simulink model "n98tot98reg57neu"  (R2023b)
settings: Solver=VariableStepAuto  StartTime=0.0  StopTime=10.0  RelTol=1e-3
libraries: neural x63
(part 2 of 3)

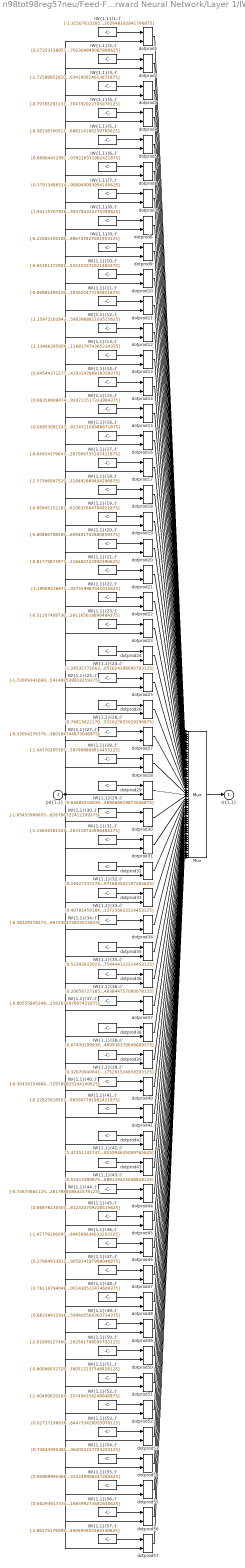
== system n98tot98reg57neu/Feed-Forward Neural Network/Layer 1/IW{1,1} ==
  "pd{1,1}" : Inport  PortDimensions=7
      mask Display: e = 0.06;c1 = [120 230 180]/255;c2 = ([120 230 180]+0)/(256+128);c3 = ([120 230 180]+128)/(256+128);patch([0 1 1 0],[0 0 1 1],c1);patch([0 1 1 1-e 1-e 0+e],[0 0 1 1-e 0+e 0+e],c2);patch([0 0 1 1-e 0+e 0+e],[0 1 1 1-e 1-e 0+e],c3);plot([0 1 1 0 0],[0 0 1 1 0]);
  "IW{1,1}(1,:)'" : Constant  Value=[-1.31507613281385449255367348087020218372344970703125;-0.3434268124643267139362023954163305461406707763671875;-0.4055668892280188675414365206961520016193389892578125;-0.58108307602678055392431133441277779638767242431640625;-1.2280217354284930220131855094223283231258392333984375;1.168197906116284823241358026280067861080169677734375;-0.55694114732430921588246519604581408202648162841796875]
      mask Display: e = 0.06;c1 = [120 150 230]/255;c2 = ([120 150 230]+0)/383;c3 = ([120 150 230]+128)/383;patch([0 1 1 0],[0 0 1 1],c1);patch([0 1 1 1-e 1-e 0+e],[0 0 1 1-e 0+e 0+e],c2);patch([0 0 1 1-e 0+e 0+e],[0 1 1 1-e 1-e 0+e],c3);plot([0 1 1 0 0],[0 0 1 1 0]);disp('Weights');
  "IW{1,1}(10,:)'" : Constant  Value=[-0.65301172901308179863377745277830399572849273681640625;0.557094329633779583588193418108858168125152587890625;-0.84973696392753306216860664790146984159946441650390625;-0.632442901627863651725647287094034254550933837890625;0.99820207808413707883943288834416307508945465087890625;-0.8724231506525537138685422178241424262523651123046875;0.76560493245783245441771214245818555355072021484375]
      mask Display: e = 0.06;c1 = [120 150 230]/255;c2 = ([120 150 230]+0)/383;c3 = ([120 150 230]+128)/383;patch([0 1 1 0],[0 0 1 1],c1);patch([0 1 1 1-e 1-e 0+e],[0 0 1 1-e 0+e 0+e],c2);patch([0 0 1 1-e 0+e 0+e],[0 1 1 1-e 1-e 0+e],c3);plot([0 1 1 0 0],[0 0 1 1 0]);disp('Weights');
  "IW{1,1}(11,:)'" : Constant  Value=[-0.06985499326512305262593116594871389679610729217529296875;-1.55742226767316171986976769403554499149322509765625;0.61111449383935878554297005393891595304012298583984375;-0.0637891933373135600060521710474858991801738739013671875;1.12246939262949130267088548862375319004058837890625;-1.345762851134290283283689859672449529170989990234375;0.95876871436280175498012567913974635303020477294921875]
      mask Display: e = 0.06;c1 = [120 150 230]/255;c2 = ([120 150 230]+0)/383;c3 = ([120 150 230]+128)/383;patch([0 1 1 0],[0 0 1 1],c1);patch([0 1 1 1-e 1-e 0+e],[0 0 1 1-e 0+e 0+e],c2);patch([0 0 1 1-e 0+e 0+e],[0 1 1 1-e 1-e 0+e],c3);plot([0 1 1 0 0],[0 0 1 1 0]);disp('Weights');
  "IW{1,1}(12,:)'" : Constant  Value=[2.159721626433666497035801512538455426692962646484375;-1.1313148038546676499294107998139224946498870849609375;-0.66185085994261905195656936484738253057003021240234375;1.6817370764954191475482048190315254032611846923828125;-0.93077989098894853281507266729022376239299774169921875;-1.173094338058920715894828390446491539478302001953125;1.2382244436054552494397285045124590396881103515625]
      mask Display: e = 0.06;c1 = [120 150 230]/255;c2 = ([120 150 230]+0)/383;c3 = ([120 150 230]+128)/383;patch([0 1 1 0],[0 0 1 1],c1);patch([0 1 1 1-e 1-e 0+e],[0 0 1 1-e 0+e 0+e],c2);patch([0 0 1 1-e 0+e 0+e],[0 1 1 1-e 1-e 0+e],c3);plot([0 1 1 0 0],[0 0 1 1 0]);disp('Weights');
  "IW{1,1}(13,:)'" : Constant  Value=[2.134962850094378250531690355273894965648651123046875;0.1810173913040981352740033116788254119455814361572265625;0.1268442563962487723561167740626842714846134185791015625;2.077238884587504497147847359883598983287811279296875;-0.03626682177452443534004800085313036106526851654052734375;-1.7725082910032003979949877248145639896392822265625;0.597079894289870960477628614171408116817474365234375]
      mask Display: e = 0.06;c1 = [120 150 230]/255;c2 = ([120 150 230]+0)/383;c3 = ([120 150 230]+128)/383;patch([0 1 1 0],[0 0 1 1],c1);patch([0 1 1 1-e 1-e 0+e],[0 0 1 1-e 0+e 0+e],c2);patch([0 0 1 1-e 0+e 0+e],[0 1 1 1-e 1-e 0+e],c3);plot([0 1 1 0 0],[0 0 1 1 0]);disp('Weights');
  "IW{1,1}(14,:)'" : Constant  Value=[0.945442711778084809992606096784584224224090576171875;-0.0565352619944564926957042416688636876642704010009765625;0.91502969793743405002572899320512078702449798583984375;-1.3291403247332258530377657734788954257965087890625;-0.71424304769140800619453557374072261154651641845703125;1.440252227385283134708515717647969722747802734375;-0.31626437150536046427617975496104918420314788818359375]
      mask Display: e = 0.06;c1 = [120 150 230]/255;c2 = ([120 150 230]+0)/383;c3 = ([120 150 230]+128)/383;patch([0 1 1 0],[0 0 1 1],c1);patch([0 1 1 1-e 1-e 0+e],[0 0 1 1-e 0+e 0+e],c2);patch([0 0 1 1-e 0+e 0+e],[0 1 1 1-e 1-e 0+e],c3);plot([0 1 1 0 0],[0 0 1 1 0]);disp('Weights');
  "IW{1,1}(15,:)'" : Constant  Value=[0.9635960847448152843952584589715115725994110107421875;0.09980816968357765495145628165118978358805179595947265625;-0.50121653240937102946617187626543454825878143310546875;-1.919415213736128666965896627516485750675201416015625;0.47845586929562278211136572281247936189174652099609375;0.941812528879230281830814419663511216640472412109375;-0.86980200940910579188170004272251389920711517333984375]
      mask Display: e = 0.06;c1 = [120 150 230]/255;c2 = ([120 150 230]+0)/383;c3 = ([120 150 230]+128)/383;patch([0 1 1 0],[0 0 1 1],c1);patch([0 1 1 1-e 1-e 0+e],[0 0 1 1-e 0+e 0+e],c2);patch([0 0 1 1-e 0+e 0+e],[0 1 1 1-e 1-e 0+e],c3);plot([0 1 1 0 0],[0 0 1 1 0]);disp('Weights');
  "IW{1,1}(16,:)'" : Constant  Value=[0.0085309114777282722685836091613964526914060115814208984375;0.76963678008214742032322419618139974772930145263671875;0.633935904479372869246844857116229832172393798828125;-0.459413204321313883848887371641467325389385223388671875;-2.435905516746778243231119631673209369182586669921875;0.77012835966411830046496334034600295126438140869140625;-0.484808047650836015929343147945473901927471160888671875]
      mask Display: e = 0.06;c1 = [120 150 230]/255;c2 = ([120 150 230]+0)/383;c3 = ([120 150 230]+128)/383;patch([0 1 1 0],[0 0 1 1],c1);patch([0 1 1 1-e 1-e 0+e],[0 0 1 1-e 0+e 0+e],c2);patch([0 0 1 1-e 0+e 0+e],[0 1 1 1-e 1-e 0+e],c3);plot([0 1 1 0 0],[0 0 1 1 0]);disp('Weights');
  "IW{1,1}(17,:)'" : Constant  Value=[-0.64954379643572435210074900169274769723415374755859375;0.5455804121247702642705235120956785976886749267578125;-1.5634615988825759647085078540840186178684234619140625;-0.84212075753120385623873289659968577325344085693359375;0.5360456525378729519815124149317853152751922607421875;-1.4042701008338334123237700623576529324054718017578125;0.21773378780089636119754459286923520267009735107421875]
      mask Display: e = 0.06;c1 = [120 150 230]/255;c2 = ([120 150 230]+0)/383;c3 = ([120 150 230]+128)/383;patch([0 1 1 0],[0 0 1 1],c1);patch([0 1 1 1-e 1-e 0+e],[0 0 1 1-e 0+e 0+e],c2);patch([0 0 1 1-e 0+e 0+e],[0 1 1 1-e 1-e 0+e],c3);plot([0 1 1 0 0],[0 0 1 1 0]);disp('Weights');
  "IW{1,1}(18,:)'" : Constant  Value=[-1.575660475296334350758797882008366286754608154296875;1.8425130461237986256861631773062981665134429931640625;0.781192060847692548719578553573228418827056884765625;1.09892397924112827922726864926517009735107421875;-0.976082267335859565804412341094575822353363037109375;-0.6852967127598470487015447361045517027378082275390625;-0.71498884111504767968625628782319836318492889404296875]
      mask Display: e = 0.06;c1 = [120 150 230]/255;c2 = ([120 150 230]+0)/383;c3 = ([120 150 230]+128)/383;patch([0 1 1 0],[0 0 1 1],c1);patch([0 1 1 1-e 1-e 0+e],[0 0 1 1-e 0+e 0+e],c2);patch([0 0 1 1-e 0+e 0+e],[0 1 1 1-e 1-e 0+e],c3);plot([0 1 1 0 0],[0 0 1 1 0]);disp('Weights');
  "IW{1,1}(19,:)'" : Constant  Value=[-0.9594515218334020989487953556817956268787384033203125;-0.48829379470511657945763772659120149910449981689453125;0.4757457278855803384232103780959732830524444580078125;0.9005439753059005791868685264489613473415374755859375;-1.0185701269266511648226014585816301405429840087890625;-1.4773529160647649316473462022258900105953216552734375;-0.726355990881138335879541045869700610637664794921875]
      mask Display: e = 0.06;c1 = [120 150 230]/255;c2 = ([120 150 230]+0)/383;c3 = ([120 150 230]+128)/383;patch([0 1 1 0],[0 0 1 1],c1);patch([0 1 1 1-e 1-e 0+e],[0 0 1 1-e 0+e 0+e],c2);patch([0 0 1 1-e 0+e 0+e],[0 1 1 1-e 1-e 0+e],c3);plot([0 1 1 0 0],[0 0 1 1 0]);disp('Weights');
  "IW{1,1}(2,:)'" : Constant  Value=[0.272531380514197840714274434503749944269657135009765625;1.0968943883890844848139067835290916264057159423828125;-0.34251944384713095548278261048835702240467071533203125;-0.874463157238554611438985375571064651012420654296875;0.9507141217692856027809966690256260335445404052734375;-0.24034301968930471549157346089486964046955108642578125;1.6368628806959615307192734690033830702304840087890625]
      mask Display: e = 0.06;c1 = [120 150 230]/255;c2 = ([120 150 230]+0)/383;c3 = ([120 150 230]+128)/383;patch([0 1 1 0],[0 0 1 1],c1);patch([0 1 1 1-e 1-e 0+e],[0 0 1 1-e 0+e 0+e],c2);patch([0 0 1 1-e 0+e 0+e],[0 1 1 1-e 1-e 0+e],c3);plot([0 1 1 0 0],[0 0 1 1 0]);disp('Weights');
  "IW{1,1}(20,:)'" : Constant  Value=[-0.8088679858537386468952945506316609680652618408203125;0.11185596548077370027129973095725290477275848388671875;1.026306998840350814816702040843665599822998046875;-0.2193307597737976510909874150456744246184825897216796875;0.96539895136091613547790757365874014794826507568359375;-1.611240681871787483459002032759599387645721435546875;0.1380372426352799164472884285714826546609401702880859375]
      mask Display: e = 0.06;c1 = [120 150 230]/255;c2 = ([120 150 230]+0)/383;c3 = ([120 150 230]+128)/383;patch([0 1 1 0],[0 0 1 1],c1);patch([0 1 1 1-e 1-e 0+e],[0 0 1 1-e 0+e 0+e],c2);patch([0 0 1 1-e 0+e 0+e],[0 1 1 1-e 1-e 0+e],c3);plot([0 1 1 0 0],[0 0 1 1 0]);disp('Weights');
  "IW{1,1}(21,:)'" : Constant  Value=[-0.8177987397310102490877170566818676888942718505859375;-0.3905060399106281554537645206437446177005767822265625;0.11055547284934041929460590836242772638797760009765625;0.1052993247470589144310082474476075731217861175537109375;-1.2126110654717712211692060009227134287357330322265625;0.607129439275836180200940361828543245792388916015625;-2.50415210712362412692755242460407316684722900390625]
      mask Display: e = 0.06;c1 = [120 150 230]/255;c2 = ([120 150 230]+0)/383;c3 = ([120 150 230]+128)/383;patch([0 1 1 0],[0 0 1 1],c1);patch([0 1 1 1-e 1-e 0+e],[0 0 1 1-e 0+e 0+e],c2);patch([0 0 1 1-e 0+e 0+e],[0 1 1 1-e 1-e 0+e],c3);plot([0 1 1 0 0],[0 0 1 1 0]);disp('Weights');
  "IW{1,1}(22,:)'" : Constant  Value=[1.19089226971850781211514913593418896198272705078125;1.45385364381177151216206766548566520214080810546875;-0.601277074598317806675140673178248107433319091796875;-0.475071026226747961107577111761202104389667510986328125;1.1590060828883947952050448293448425829410552978515625;-0.223577539094418853427015392298926599323749542236328125;0.52854958185949441062945197700173594057559967041015625]
      mask Display: e = 0.06;c1 = [120 150 230]/255;c2 = ([120 150 230]+0)/383;c3 = ([120 150 230]+128)/383;patch([0 1 1 0],[0 0 1 1],c1);patch([0 1 1 1-e 1-e 0+e],[0 0 1 1-e 0+e 0+e],c2);patch([0 0 1 1-e 0+e 0+e],[0 1 1 1-e 1-e 0+e],c3);plot([0 1 1 0 0],[0 0 1 1 0]);disp('Weights');
  "IW{1,1}(23,:)'" : Constant  Value=[-0.51107408730064118884683921351097524166107177734375;-0.69542516098775897237516119275824166834354400634765625;-1.4905003550878583862271398174925707280635833740234375;1.0412183770694818374380474779172800481319427490234375;-0.858888834537086420795048979925923049449920654296875;0.126966453545523716428533589350990951061248779296875;-0.879111162983166050111094591557048261165618896484375]
      mask Display: e = 0.06;c1 = [120 150 230]/255;c2 = ([120 150 230]+0)/383;c3 = ([120 150 230]+128)/383;patch([0 1 1 0],[0 0 1 1],c1);patch([0 1 1 1-e 1-e 0+e],[0 0 1 1-e 0+e 0+e],c2);patch([0 0 1 1-e 0+e 0+e],[0 1 1 1-e 1-e 0+e],c3);plot([0 1 1 0 0],[0 0 1 1 0]);disp('Weights');
  "IW{1,1}(24,:)'" : Constant  Value=[1.2453577166389904196108773248852230608463287353515625;-0.242279955231003818472146349449758417904376983642578125;-0.6152732028289682464361476377234794199466705322265625;-0.52848261741762225796037455438636243343353271484375;-1.3356713480763762191827481728978455066680908203125;-0.7798150291085292895587599559803493320941925048828125;1.316557903300858090034353153896518051624298095703125]
      mask Display: e = 0.06;c1 = [120 150 230]/255;c2 = ([120 150 230]+0)/383;c3 = ([120 150 230]+128)/383;patch([0 1 1 0],[0 0 1 1],c1);patch([0 1 1 1-e 1-e 0+e],[0 0 1 1-e 0+e 0+e],c2);patch([0 0 1 1-e 0+e 0+e],[0 1 1 1-e 1-e 0+e],c3);plot([0 1 1 0 0],[0 0 1 1 0]);disp('Weights');
  "IW{1,1}(25,:)'" : Constant  Value=[-1.720093416906787187059535426669754087924957275390625;-1.1755779750190813448540438912459649145603179931640625;-0.273381324463259745005672129991580732166767120361328125;0.92851119014197058820769825615570880472660064697265625;0.78830859911427586528276378885493613779544830322265625;0.53710877686837321665080935417790897190570831298828125;-0.0931050198316623889294163518570712767541408538818359375]
      mask Display: e = 0.06;c1 = [120 150 230]/255;c2 = ([120 150 230]+0)/383;c3 = ([120 150 230]+128)/383;patch([0 1 1 0],[0 0 1 1],c1);patch([0 1 1 1-e 1-e 0+e],[0 0 1 1-e 0+e 0+e],c2);patch([0 0 1 1-e 0+e 0+e],[0 1 1 1-e 1-e 0+e],c3);plot([0 1 1 0 0],[0 0 1 1 0]);disp('Weights');
  "IW{1,1}(26,:)'" : Constant  Value=[0.7681562217053945484934729392989538609981536865234375;1.3209871255882330576270078381639905273914337158203125;-0.495847608712504717143332300111069343984127044677734375;-0.768492213819274905262091124313883483409881591796875;1.4607032300264208846130031815846450626850128173828125;1.4314160847875883053603729422320611774921417236328125;0.63011690839067202585255245139705948531627655029296875]
      mask Display: e = 0.06;c1 = [120 150 230]/255;c2 = ([120 150 230]+0)/383;c3 = ([120 150 230]+128)/383;patch([0 1 1 0],[0 0 1 1],c1);patch([0 1 1 1-e 1-e 0+e],[0 0 1 1-e 0+e 0+e],c2);patch([0 0 1 1-e 0+e 0+e],[0 1 1 1-e 1-e 0+e],c3);plot([0 1 1 0 0],[0 0 1 1 0]);disp('Weights');
  "IW{1,1}(27,:)'" : Constant  Value=[-0.330542763766594027696754665157641284167766571044921875;1.4209623056183582345823879222734831273555755615234375;-1.3540278759723431978301277922582812607288360595703125;1.239950698517690685918068993487395346164703369140625;0.244622420985858901598675174682284705340862274169921875;-0.69335046389705023983651699381880462169647216796875;0.04286899583435747895787670813660952262580394744873046875]
      mask Display: e = 0.06;c1 = [120 150 230]/255;c2 = ([120 150 230]+0)/383;c3 = ([120 150 230]+128)/383;patch([0 1 1 0],[0 0 1 1],c1);patch([0 1 1 1-e 1-e 0+e],[0 0 1 1-e 0+e 0+e],c2);patch([0 0 1 1-e 0+e 0+e],[0 1 1 1-e 1-e 0+e],c3);plot([0 1 1 0 0],[0 0 1 1 0]);disp('Weights');
  "IW{1,1}(28,:)'" : Constant  Value=[-1.44370205397184481199701622244901955127716064453125;0.483062098703527009746494513819925487041473388671875;0.325262798677855291540339521816349588334560394287109375;1.87353161972341819563325771014206111431121826171875;-0.469898365036419407569923123446642421185970306396484375;-0.52795627331928962622242806901340372860431671142578125;-0.6150982768929271760072197139379568397998809814453125]
      mask Display: e = 0.06;c1 = [120 150 230]/255;c2 = ([120 150 230]+0)/383;c3 = ([120 150 230]+128)/383;patch([0 1 1 0],[0 0 1 1],c1);patch([0 1 1 1-e 1-e 0+e],[0 0 1 1-e 0+e 0+e],c2);patch([0 0 1 1-e 0+e 0+e],[0 1 1 1-e 1-e 0+e],c3);plot([0 1 1 0 0],[0 0 1 1 0]);disp('Weights');
  "IW{1,1}(29,:)'" : Constant  Value=[0.64685516039214252526079462768393568694591522216796875;-0.7133517745537172327630059953662566840648651123046875;-1.1162505593597875641620476017124019563198089599609375;1.4296859613759911322716789072728715837001800537109375;-1.673504671100669582983755390159785747528076171875;-0.2356418802824417346730712097269133664667606353759765625;0.1731214195331098604224706605236860923469066619873046875]
      mask Display: e = 0.06;c1 = [120 150 230]/255;c2 = ([120 150 230]+0)/383;c3 = ([120 150 230]+128)/383;patch([0 1 1 0],[0 0 1 1],c1);patch([0 1 1 1-e 1-e 0+e],[0 0 1 1-e 0+e 0+e],c2);patch([0 0 1 1-e 0+e 0+e],[0 1 1 1-e 1-e 0+e],c3);plot([0 1 1 0 0],[0 0 1 1 0]);disp('Weights');
  "IW{1,1}(3,:)'" : Constant  Value=[-1.7258895161045704202962269846466369926929473876953125;-0.96905544802317578056971569822053425014019012451171875;-0.2467907702150093085524673597319633699953556060791015625;0.620713226509980398049037830787710845470428466796875;-0.58216038095865296764230834014597348868846893310546875;0.8234144012332003104148725469713099300861358642578125;0.69431564257952060881251554746995680034160614013671875]
      mask Display: e = 0.06;c1 = [120 150 230]/255;c2 = ([120 150 230]+0)/383;c3 = ([120 150 230]+128)/383;patch([0 1 1 0],[0 0 1 1],c1);patch([0 1 1 1-e 1-e 0+e],[0 0 1 1-e 0+e 0+e],c2);patch([0 0 1 1-e 0+e 0+e],[0 1 1 1-e 1-e 0+e],c3);plot([0 1 1 0 0],[0 0 1 1 0]);disp('Weights');
  "IW{1,1}(30,:)'" : Constant  Value=[-1.05455966655188593250613848795183002948760986328125;0.627223375235642865987983896047808229923248291015625;0.12537337491597810856802652779151685535907745361328125;0.2444653558883956023795036571755190379917621612548828125;-0.66100938577782974991947639864520169794559478759765625;-0.360249769337874337082894271588884294033050537109375;1.6012452229692220040391248403466306626796722412109375]
      mask Display: e = 0.06;c1 = [120 150 230]/255;c2 = ([120 150 230]+0)/383;c3 = ([120 150 230]+128)/383;patch([0 1 1 0],[0 0 1 1],c1);patch([0 1 1 1-e 1-e 0+e],[0 0 1 1-e 0+e 0+e],c2);patch([0 0 1 1-e 0+e 0+e],[0 1 1 1-e 1-e 0+e],c3);plot([0 1 1 0 0],[0 0 1 1 0]);disp('Weights');
  "IW{1,1}(31,:)'" : Constant  Value=[-1.1563458134754280859368691380950622260570526123046875;-0.93459383751556490693701562122441828250885009765625;-1.3360775871392422953221057468908838927745819091796875;0.0993024254056518451694302029864047653973102569580078125;0.00133754034631904106245059438151656650006771087646484375;-0.67390772930921460925901556038297712802886962890625;-1.3895944435588647447588073191582225263118743896484375]
      mask Display: e = 0.06;c1 = [120 150 230]/255;c2 = ([120 150 230]+0)/383;c3 = ([120 150 230]+128)/383;patch([0 1 1 0],[0 0 1 1],c1);patch([0 1 1 1-e 1-e 0+e],[0 0 1 1-e 0+e 0+e],c2);patch([0 0 1 1-e 0+e 0+e],[0 1 1 1-e 1-e 0+e],c3);plot([0 1 1 0 0],[0 0 1 1 0]);disp('Weights');
  "IW{1,1}(32,:)'" : Constant  Value=[0.164273372784759341680427269238862209022045135498046875;0.33065648688842308455804186451132409274578094482421875;-1.0794971677089122419346267633954994380474090576171875;-0.7715801043565042593996849973336793482303619384765625;2.13032359300715246064328312058933079242706298828125;-0.67381390592311607434794495929963886737823486328125;-0.416767412004134973901869898327277041971683502197265625]
      mask Display: e = 0.06;c1 = [120 150 230]/255;c2 = ([120 150 230]+0)/383;c3 = ([120 150 230]+128)/383;patch([0 1 1 0],[0 0 1 1],c1);patch([0 1 1 1-e 1-e 0+e],[0 0 1 1-e 0+e 0+e],c2);patch([0 0 1 1-e 0+e 0+e],[0 1 1 1-e 1-e 0+e],c3);plot([0 1 1 0 0],[0 0 1 1 0]);disp('Weights');
  "IW{1,1}(33,:)'" : Constant  Value=[0.4078145918403646152938790692132897675037384033203125;-0.25400961624534179605916506261564791202545166015625;0.299496744344248444491540794842876493930816650390625;-1.315968686900561568364764752914197742938995361328125;0.354585810747044816171325010145665146410465240478515625;-1.5340931197175560196654942046734504401683807373046875;-1.1679631626616970851983978718635626137256622314453125]
      mask Display: e = 0.06;c1 = [120 150 230]/255;c2 = ([120 150 230]+0)/383;c3 = ([120 150 230]+128)/383;patch([0 1 1 0],[0 0 1 1],c1);patch([0 1 1 1-e 1-e 0+e],[0 0 1 1-e 0+e 0+e],c2);patch([0 0 1 1-e 0+e 0+e],[0 1 1 1-e 1-e 0+e],c3);plot([0 1 1 0 0],[0 0 1 1 0]);disp('Weights');
  "IW{1,1}(34,:)'" : Constant  Value=[-0.383293782731273513508796213500318117439746856689453125;-0.49477857434749916709648687174194492399692535400390625;1.0735125951492159313005458898260258138179779052734375;-0.356137381639198558058723165231640450656414031982421875;0.8366603229741580438627579496824182569980621337890625;1.1696293190818807250508370998431928455829620361328125;0.82042281814013462426515843617380596697330474853515625]
      mask Display: e = 0.06;c1 = [120 150 230]/255;c2 = ([120 150 230]+0)/383;c3 = ([120 150 230]+128)/383;patch([0 1 1 0],[0 0 1 1],c1);patch([0 1 1 1-e 1-e 0+e],[0 0 1 1-e 0+e 0+e],c2);patch([0 0 1 1-e 0+e 0+e],[0 1 1 1-e 1-e 0+e],c3);plot([0 1 1 0 0],[0 0 1 1 0]);disp('Weights');
  "IW{1,1}(35,:)'" : Constant  Value=[0.52342833023374002454630726788309402763843536376953125;0.6610984420440237929739168976084329187870025634765625;-1.56739612395232796870914171449840068817138671875;-0.10778307833886487110408580747389351017773151397705078125;1.48495649719330646831849662703461945056915283203125;-0.57665955778967836753423625850700773298740386962890625;-0.043990733229857033326215542956560966558754444122314453125]
      mask Display: e = 0.06;c1 = [120 150 230]/255;c2 = ([120 150 230]+0)/383;c3 = ([120 150 230]+128)/383;patch([0 1 1 0],[0 0 1 1],c1);patch([0 1 1 1-e 1-e 0+e],[0 0 1 1-e 0+e 0+e],c2);patch([0 0 1 1-e 0+e 0+e],[0 1 1 1-e 1-e 0+e],c3);plot([0 1 1 0 0],[0 0 1 1 0]);disp('Weights');
  "IW{1,1}(36,:)'" : Constant  Value=[0.2065672716597789226877779356073006056249141693115234375;0.08562058777203361559227090538115589879453182220458984375;-0.67599687037562450342420561355538666248321533203125;1.365395669432860170644516983884386718273162841796875;0.80146873586901679065164216808625496923923492431640625;0.74085208226540755216404932070872746407985687255859375;-1.311866403168686634472805963014252483844757080078125]
      mask Display: e = 0.06;c1 = [120 150 230]/255;c2 = ([120 150 230]+0)/383;c3 = ([120 150 230]+128)/383;patch([0 1 1 0],[0 0 1 1],c1);patch([0 1 1 1-e 1-e 0+e],[0 0 1 1-e 0+e 0+e],c2);patch([0 0 1 1-e 0+e 0+e],[0 1 1 1-e 1-e 0+e],c3);plot([0 1 1 0 0],[0 0 1 1 0]);disp('Weights');
  "IW{1,1}(37,:)'" : Constant  Value=[-0.0055584524497600505676953019928987487219274044036865234375;0.1283486422105139801441708868878777138888835906982421875;0.64246359209079317853507973268278874456882476806640625;2.373547021175534954551267219358123838901519775390625;-0.65169536182719145500641388935036957263946533203125;-1.2696853941598613690899810535483993589878082275390625;0.247748997273591065049203052694792859256267547607421875]
      mask Display: e = 0.06;c1 = [120 150 230]/255;c2 = ([120 150 230]+0)/383;c3 = ([120 150 230]+128)/383;patch([0 1 1 0],[0 0 1 1],c1);patch([0 1 1 1-e 1-e 0+e],[0 0 1 1-e 0+e 0+e],c2);patch([0 0 1 1-e 0+e 0+e],[0 1 1 1-e 1-e 0+e],c3);plot([0 1 1 0 0],[0 0 1 1 0]);disp('Weights');
  "IW{1,1}(38,:)'" : Constant  Value=[0.6743029993834757096493603967246599495410919189453125;1.2825796750331457385385647285147570073604583740234375;0.0790396474226212342184538783840253017842769622802734375;-1.2783619596419928399200216517783701419830322265625;-0.18957683849344919568835621248581446707248687744140625;-1.2988703840486512941510000018752180039882659912109375;-1.775056455486147655165041214786469936370849609375]
      mask Display: e = 0.06;c1 = [120 150 230]/255;c2 = ([120 150 230]+0)/383;c3 = ([120 150 230]+128)/383;patch([0 1 1 0],[0 0 1 1],c1);patch([0 1 1 1-e 1-e 0+e],[0 0 1 1-e 0+e 0+e],c2);patch([0 0 1 1-e 0+e 0+e],[0 1 1 1-e 1-e 0+e],c3);plot([0 1 1 0 0],[0 0 1 1 0]);disp('Weights');
  "IW{1,1}(39,:)'" : Constant  Value=[0.32070940641117962055517409680760465562343597412109375;-0.302884329744402436279671064767171628773212432861328125;-0.70135171405963225854662823621765710413455963134765625;-0.2032094030910858439842314737688866443932056427001953125;-1.9486140255028499002065700551611371338367462158203125;0.6282895046964067642392137713613919913768768310546875;0.136779552133337756192332790305954404175281524658203125]
      mask Display: e = 0.06;c1 = [120 150 230]/255;c2 = ([120 150 230]+0)/383;c3 = ([120 150 230]+128)/383;patch([0 1 1 0],[0 0 1 1],c1);patch([0 1 1 1-e 1-e 0+e],[0 0 1 1-e 0+e 0+e],c2);patch([0 0 1 1-e 0+e 0+e],[0 1 1 1-e 1-e 0+e],c3);plot([0 1 1 0 0],[0 0 1 1 0]);disp('Weights');
  "IW{1,1}(4,:)'" : Constant  Value=[-0.7978529313140108047974763394449837505817413330078125;1.0539972191159165948448617200483568012714385986328125;-1.0799823570469537781235658258083276450634002685546875;0.0668246115812050345272865570223075337707996368408203125;-0.267165552329517497209820930947898887097835540771484375;1.4805124907494973118815551060833968222141265869140625;1.470672904788721258029227101360447704792022705078125]
      mask Display: e = 0.06;c1 = [120 150 230]/255;c2 = ([120 150 230]+0)/383;c3 = ([120 150 230]+128)/383;patch([0 1 1 0],[0 0 1 1],c1);patch([0 1 1 1-e 1-e 0+e],[0 0 1 1-e 0+e 0+e],c2);patch([0 0 1 1-e 0+e 0+e],[0 1 1 1-e 1-e 0+e],c3);plot([0 1 1 0 0],[0 0 1 1 0]);disp('Weights');
  "IW{1,1}(40,:)'" : Constant  Value=[-0.3043415488474756624981409913743846118450164794921875;-0.348329945045467381792292371756047941744327545166015625;1.4245644902585041791098774410784244537353515625;0.59723849123039529640522005138336680829524993896484375;-0.95038484958970415039658519162912853062152862548828125;1.6222299863679292553086952466401271522045135498046875;-0.68245442425327740298968137722113169729709625244140625]
      mask Display: e = 0.06;c1 = [120 150 230]/255;c2 = ([120 150 230]+0)/383;c3 = ([120 150 230]+128)/383;patch([0 1 1 0],[0 0 1 1],c1);patch([0 1 1 1-e 1-e 0+e],[0 0 1 1-e 0+e 0+e],c2);patch([0 0 1 1-e 0+e 0+e],[0 1 1 1-e 1-e 0+e],c3);plot([0 1 1 0 0],[0 0 1 1 0]);disp('Weights');
  "IW{1,1}(41,:)'" : Constant  Value=[-0.228250185520216530843384816762409172952175140380859375;1.107167413982370618441564147360622882843017578125;-0.9640363396052424871385255755740217864513397216796875;-0.0840881104006174495690828507576952688395977020263671875;-1.415538736015257814671031155739910900592803955078125;-0.84324168186591286211495344105060212314128875732421875;-1.7168224195788972519238768654759041965007781982421875]
      mask Display: e = 0.06;c1 = [120 150 230]/255;c2 = ([120 150 230]+0)/383;c3 = ([120 150 230]+128)/383;patch([0 1 1 0],[0 0 1 1],c1);patch([0 1 1 1-e 1-e 0+e],[0 0 1 1-e 0+e 0+e],c2);patch([0 0 1 1-e 0+e 0+e],[0 1 1 1-e 1-e 0+e],c3);plot([0 1 1 0 0],[0 0 1 1 0]);disp('Weights');
  "IW{1,1}(42,:)'" : Constant  Value=[1.4155114274714801769761152172577567398548126220703125;1.3239165256278895288488683945615775883197784423828125;-1.3501203682438500663920422084629535675048828125;0.2328620769492155684332601595087908208370208740234375;0.55894536772878733454916755363228730857372283935546875;0.0407950042051287986577534638854558579623699188232421875;-1.0232721669545858933503268417553044855594635009765625]
      mask Display: e = 0.06;c1 = [120 150 230]/255;c2 = ([120 150 230]+0)/383;c3 = ([120 150 230]+128)/383;patch([0 1 1 0],[0 0 1 1],c1);patch([0 1 1 1-e 1-e 0+e],[0 0 1 1-e 0+e 0+e],c2);patch([0 0 1 1-e 0+e 0+e],[0 1 1 1-e 1-e 0+e],c3);plot([0 1 1 0 0],[0 0 1 1 0]);disp('Weights');
  "IW{1,1}(43,:)'" : Constant  Value=[0.55413390875951951120015337437507696449756622314453125;1.4175262241961592568628702792921103537082672119140625;1.2748511369893245070983311961754225194454193115234375;-1.182494040136969459808824467472732067108154296875;-0.58114960985459107600803463355987332761287689208984375;-0.857972175702311989908821487915702164173126220703125;0.92870706770252653416974908395786769688129425048828125]
      mask Display: e = 0.06;c1 = [120 150 230]/255;c2 = ([120 150 230]+0)/383;c3 = ([120 150 230]+128)/383;patch([0 1 1 0],[0 0 1 1],c1);patch([0 1 1 1-e 1-e 0+e],[0 0 1 1-e 0+e 0+e],c2);patch([0 0 1 1-e 0+e 0+e],[0 1 1 1-e 1-e 0+e],c3);plot([0 1 1 0 0],[0 0 1 1 0]);disp('Weights');
  "IW{1,1}(44,:)'" : Constant  Value=[-0.726738611258897382327859304496087133884429931640625;1.4637246388394091756168791107484139502048492431640625;-1.201506697000127577013017798890359699726104736328125;-0.81251968811314434493198177733574993908405303955078125;-0.8625314523673370814549343776889145374298095703125;-1.6996062115963062044698972385958768427371978759765625;-1.924622498805697023982475002412684261798858642578125]
      mask Display: e = 0.06;c1 = [120 150 230]/255;c2 = ([120 150 230]+0)/383;c3 = ([120 150 230]+128)/383;patch([0 1 1 0],[0 0 1 1],c1);patch([0 1 1 1-e 1-e 0+e],[0 0 1 1-e 0+e 0+e],c2);patch([0 0 1 1-e 0+e 0+e],[0 1 1 1-e 1-e 0+e],c3);plot([0 1 1 0 0],[0 0 1 1 0]);disp('Weights');
  "IW{1,1}(45,:)'" : Constant  Value=[0.80676130501258003224762660465785302221775054931640625;-0.34224277670567471165696815660339780151844024658203125;-1.2528533394914862508784381134319119155406951904296875;0.50145991018622348978084346526884473860263824462890625;1.0931712551173531355885870652855373919010162353515625;-1.19258240643649582324314906145446002483367919921875;1.015863450240984011685441146255470812320709228515625]
      mask Display: e = 0.06;c1 = [120 150 230]/255;c2 = ([120 150 230]+0)/383;c3 = ([120 150 230]+128)/383;patch([0 1 1 0],[0 0 1 1],c1);patch([0 1 1 1-e 1-e 0+e],[0 0 1 1-e 0+e 0+e],c2);patch([0 0 1 1-e 0+e 0+e],[0 1 1 1-e 1-e 0+e],c3);plot([0 1 1 0 0],[0 0 1 1 0]);disp('Weights');
  "IW{1,1}(46,:)'" : Constant  Value=[-1.47779106095812462484673233120702207088470458984375;-1.122888888551688335581957289832644164562225341796875;0.028169618732438894692649000717210583388805389404296875;1.0543478201684128858772737658000551164150238037109375;0.51140915802358477559863558781216852366924285888671875;1.2389005852638106386365279831807129085063934326171875;0.582246808451106545589937013573944568634033203125]
      mask Display: e = 0.06;c1 = [120 150 230]/255;c2 = ([120 150 230]+0)/383;c3 = ([120 150 230]+128)/383;patch([0 1 1 0],[0 0 1 1],c1);patch([0 1 1 1-e 1-e 0+e],[0 0 1 1-e 0+e 0+e],c2);patch([0 0 1 1-e 0+e 0+e],[0 1 1 1-e 1-e 0+e],c3);plot([0 1 1 0 0],[0 0 1 1 0]);disp('Weights');
  "IW{1,1}(47,:)'" : Constant  Value=[0.278846138129484000245383867877535521984100341796875;0.5421300258783949832519510891870595514774322509765625;1.520332276502161850118000074871815741062164306640625;3.250848634646732904229793348349630832672119140625;-1.3936441538131052464422054981696419417858123779296875;-0.967748366202124454815702847554348409175872802734375;0.98485882175750727451912780452403239905834197998046875]
      mask Display: e = 0.06;c1 = [120 150 230]/255;c2 = ([120 150 230]+0)/383;c3 = ([120 150 230]+128)/383;patch([0 1 1 0],[0 0 1 1],c1);patch([0 1 1 1-e 1-e 0+e],[0 0 1 1-e 0+e 0+e],c2);patch([0 0 1 1-e 0+e 0+e],[0 1 1 1-e 1-e 0+e],c3);plot([0 1 1 0 0],[0 0 1 1 0]);disp('Weights');
  "IW{1,1}(48,:)'" : Constant  Value=[0.76110794048341523510003980845795013010501861572265625;0.57039260443123518395935889202519319951534271240234375;-1.368883984680971277470007407828234136104583740234375;0.67921665567346389824621155639761127531528472900390625;1.3023096880356075377704883067053742706775665283203125;-0.7905634187083998565270803737803362309932708740234375;0.6992233312007305467972173573798500001430511474609375]
      mask Display: e = 0.06;c1 = [120 150 230]/255;c2 = ([120 150 230]+0)/383;c3 = ([120 150 230]+128)/383;patch([0 1 1 0],[0 0 1 1],c1);patch([0 1 1 1-e 1-e 0+e],[0 0 1 1-e 0+e 0+e],c2);patch([0 0 1 1-e 0+e 0+e],[0 1 1 1-e 1-e 0+e],c3);plot([0 1 1 0 0],[0 0 1 1 0]);disp('Weights');
  "IW{1,1}(49,:)'" : Constant  Value=[0.8623841293628105031388031420647166669368743896484375;-0.97472812855899160222605814851704053580760955810546875;0.1192423535185637983868645051188650541007518768310546875;-1.486369120151858513878551093512214720249176025390625;-0.268964697498312421686250672792084515094757080078125;1.2233764580472084038120783588965423405170440673828125;-1.0908811533020832396090327165438793599605560302734375]
      mask Display: e = 0.06;c1 = [120 150 230]/255;c2 = ([120 150 230]+0)/383;c3 = ([120 150 230]+128)/383;patch([0 1 1 0],[0 0 1 1],c1);patch([0 1 1 1-e 1-e 0+e],[0 0 1 1-e 0+e 0+e],c2);patch([0 0 1 1-e 0+e 0+e],[0 1 1 1-e 1-e 0+e],c3);plot([0 1 1 0 0],[0 0 1 1 0]);disp('Weights');
  "IW{1,1}(5,:)'" : Constant  Value=[-0.58138790511689253381888420335599221289157867431640625;-0.65880063345359196613770791373099200427532196044921875;1.4096042047214663028853465220890939235687255859375;0.34486942223569638787949998004478402435779571533203125;-1.4203072312962792267398981493897736072540283203125;0.409729931375787892466888706621830351650714874267578125;-1.041157766591116029530894593335688114166259765625]
      mask Display: e = 0.06;c1 = [120 150 230]/255;c2 = ([120 150 230]+0)/383;c3 = ([120 150 230]+128)/383;patch([0 1 1 0],[0 0 1 1],c1);patch([0 1 1 1-e 1-e 0+e],[0 0 1 1-e 0+e 0+e],c2);patch([0 0 1 1-e 0+e 0+e],[0 1 1 1-e 1-e 0+e],c3);plot([0 1 1 0 0],[0 0 1 1 0]);disp('Weights');
  "IW{1,1}(50,:)'" : Constant  Value=[-2.0100912746005459297293782583437860012054443359375;0.538667629236171396911458941758610308170318603515625;0.8460442996788934966190254272078163921833038330078125;0.54672636157000076284617762212292291224002838134765625;0.0428779124158281399470382666549994610249996185302734375;-0.3800158870698984170388712300336919724941253662109375;0.9564860283534184492992835657787509262561798095703125]
      mask Display: e = 0.06;c1 = [120 150 230]/255;c2 = ([120 150 230]+0)/383;c3 = ([120 150 230]+128)/383;patch([0 1 1 0],[0 0 1 1],c1);patch([0 1 1 1-e 1-e 0+e],[0 0 1 1-e 0+e 0+e],c2);patch([0 0 1 1-e 0+e 0+e],[0 1 1 1-e 1-e 0+e],c3);plot([0 1 1 0 0],[0 0 1 1 0]);disp('Weights');
  "IW{1,1}(51,:)'" : Constant  Value=[-0.8008603272872314438046714712982065975666046142578125;1.181813951369524939849497968680225312709808349609375;1.45341173582876859171619798871688544750213623046875;0.031643207316806302997758137962591717950999736785888671875;-1.27707297741641578880944507545791566371917724609375;0.4095551508267745166591566885472275316715240478515625;-0.54946523735455787829096152563579380512237548828125]
      mask Display: e = 0.06;c1 = [120 150 230]/255;c2 = ([120 150 230]+0)/383;c3 = ([120 150 230]+128)/383;patch([0 1 1 0],[0 0 1 1],c1);patch([0 1 1 1-e 1-e 0+e],[0 0 1 1-e 0+e 0+e],c2);patch([0 0 1 1-e 0+e 0+e],[0 1 1 1-e 1-e 0+e],c3);plot([0 1 1 0 0],[0 0 1 1 0]);disp('Weights');
  "IW{1,1}(52,:)'" : Constant  Value=[-1.4049961910448309776455744213308207690715789794921875;0.62233100522147555277996389122563414275646209716796875;-0.97129219302346048170448966629919596016407012939453125;0.55848844717713463925434780321666039526462554931640625;-1.1790458629617859287463943473994731903076171875;0.81200884306482612462474435233161784708499908447265625;-1.485467988039626430207817975315265357494354248046875]
      mask Display: e = 0.06;c1 = [120 150 230]/255;c2 = ([120 150 230]+0)/383;c3 = ([120 150 230]+128)/383;patch([0 1 1 0],[0 0 1 1],c1);patch([0 1 1 1-e 1-e 0+e],[0 0 1 1-e 0+e 0+e],c2);patch([0 0 1 1-e 0+e 0+e],[0 1 1 1-e 1-e 0+e],c3);plot([0 1 1 0 0],[0 0 1 1 0]);disp('Weights');
  "IW{1,1}(53,:)'" : Constant  Value=[0.0273719663653070009734502576748127466998994350433349609375;0.60452433245751813206680935763870365917682647705078125;-0.342499870094015335109105535593698732554912567138671875;0.037294816683247695998648651993789826519787311553955078125;-1.9890933692998411519425872029387392103672027587890625;0.89523370265885315877341099621844477951526641845703125;-0.9596706835116197709112384472973644733428955078125]
      mask Display: e = 0.06;c1 = [120 150 230]/255;c2 = ([120 150 230]+0)/383;c3 = ([120 150 230]+128)/383;patch([0 1 1 0],[0 0 1 1],c1);patch([0 1 1 1-e 1-e 0+e],[0 0 1 1-e 0+e 0+e],c2);patch([0 0 1 1-e 0+e 0+e],[0 1 1 1-e 1-e 0+e],c3);plot([0 1 1 0 0],[0 0 1 1 0]);disp('Weights');
  "IW{1,1}(54,:)'" : Constant  Value=[0.73643095385122603335759094989043660461902618408203125;-1.7308297451524834453806533929309807717800140380859375;1.14113534185414788879597836057655513286590576171875;-0.80111469908175048093568193507962860167026519775390625;-0.023487767784544144600289428126416169106960296630859375;1.0837283417575089838891244653495959937572479248046875;0.9838086473510412321985540984314866364002227783203125]
      mask Display: e = 0.06;c1 = [120 150 230]/255;c2 = ([120 150 230]+0)/383;c3 = ([120 150 230]+128)/383;patch([0 1 1 0],[0 0 1 1],c1);patch([0 1 1 1-e 1-e 0+e],[0 0 1 1-e 0+e 0+e],c2);patch([0 0 1 1-e 0+e 0+e],[0 1 1 1-e 1-e 0+e],c3);plot([0 1 1 0 0],[0 0 1 1 0]);disp('Weights');
  "IW{1,1}(55,:)'" : Constant  Value=[0.958699953667932813772267763852141797542572021484375;1.36912315954559904440657192026264965534210205078125;-0.6673942941850723453711680122069083154201507568359375;-1.2053877734075009175995774057810194790363311767578125;-1.1076066384092759786739179617143236100673675537109375;1.0281675891500665631639321873080916702747344970703125;0.18998062635500989614456557319499552249908447265625]
      mask Display: e = 0.06;c1 = [120 150 230]/255;c2 = ([120 150 230]+0)/383;c3 = ([120 150 230]+128)/383;patch([0 1 1 0],[0 0 1 1],c1);patch([0 1 1 1-e 1-e 0+e],[0 0 1 1-e 0+e 0+e],c2);patch([0 0 1 1-e 0+e 0+e],[0 1 1 1-e 1-e 0+e],c3);plot([0 1 1 0 0],[0 0 1 1 0]);disp('Weights');
  "IW{1,1}(56,:)'" : Constant  Value=[0.60293617334203541968662420913460664451122283935546875;0.00643405257743377700929698903564712963998317718505859375;0.160338176186695491320932660528342239558696746826171875;-1.271045500456771559782964686746709048748016357421875;-0.06239920260555513464861832062524626962840557098388671875;-0.89147008356325774247608251243946142494678497314453125;-0.55046970433886033280401761658140458166599273681640625]
      mask Display: e = 0.06;c1 = [120 150 230]/255;c2 = ([120 150 230]+0)/383;c3 = ([120 150 230]+128)/383;patch([0 1 1 0],[0 0 1 1],c1);patch([0 1 1 1-e 1-e 0+e],[0 0 1 1-e 0+e 0+e],c2);patch([0 0 1 1-e 0+e 0+e],[0 1 1 1-e 1-e 0+e],c3);plot([0 1 1 0 0],[0 0 1 1 0]);disp('Weights');
  "IW{1,1}(57,:)'" : Constant  Value=[-2.861751760994910132041013639536686241626739501953125;2.725809114304893032709742328734137117862701416015625;-0.218663204142888201175765061634592711925506591796875;-0.209566409187355640053596061989082954823970794677734375;-0.567639257122665608079614685266278684139251708984375;-0.59830837122214119982999136482249014079570770263671875;-2.435425569850553362272194135584868490695953369140625]
      mask Display: e = 0.06;c1 = [120 150 230]/255;c2 = ([120 150 230]+0)/383;c3 = ([120 150 230]+128)/383;patch([0 1 1 0],[0 0 1 1],c1);patch([0 1 1 1-e 1-e 0+e],[0 0 1 1-e 0+e 0+e],c2);patch([0 0 1 1-e 0+e 0+e],[0 1 1 1-e 1-e 0+e],c3);plot([0 1 1 0 0],[0 0 1 1 0]);disp('Weights');
  "IW{1,1}(6,:)'" : Constant  Value=[0.80964452991338797804843352423631586134433746337890625;-1.0488823731617313850250639006844721734523773193359375;-1.053854831123814950188943839748390018939971923828125;0.00057601287814430801592635589258861728012561798095703125;-0.0668263207806062686788806104232207871973514556884765625;2.097487857646931797006573106045834720134735107421875;0.97620087490688767228874667125637643039226531982421875]
      mask Display: e = 0.06;c1 = [120 150 230]/255;c2 = ([120 150 230]+0)/383;c3 = ([120 150 230]+128)/383;patch([0 1 1 0],[0 0 1 1],c1);patch([0 1 1 1-e 1-e 0+e],[0 0 1 1-e 0+e 0+e],c2);patch([0 0 1 1-e 0+e 0+e],[0 1 1 1-e 1-e 0+e],c3);plot([0 1 1 0 0],[0 0 1 1 0]);disp('Weights');
  "IW{1,1}(7,:)'" : Constant  Value=[0.379134865144659050084641194189316593110561370849609375;0.1678271527598384771362560741181368939578533172607421875;-0.99829436130849347197369070272543467581272125244140625;-0.49443294392237147061308633055887185037136077880859375;1.477926274248878346639912706450559198856353759765625;-1.398011834695039201648114612908102571964263916015625;-0.96400318272281371179133202531374990940093994140625]
      mask Display: e = 0.06;c1 = [120 150 230]/255;c2 = ([120 150 230]+0)/383;c3 = ([120 150 230]+128)/383;patch([0 1 1 0],[0 0 1 1],c1);patch([0 1 1 1-e 1-e 0+e],[0 0 1 1-e 0+e 0+e],c2);patch([0 0 1 1-e 0+e 0+e],[0 1 1 1-e 1-e 0+e],c3);plot([0 1 1 0 0],[0 0 1 1 0]);disp('Weights');
  "IW{1,1}(8,:)'" : Constant  Value=[1.9411576792659699375320769831887446343898773193359375;-0.2328024405776709659932066642795689404010772705078125;-1.92852707782663568281122934422455728054046630859375;0.00525509251571039566475196380679335561580955982208251953125;0.307945256038169024037642884650267660617828369140625;0.1061122674367058760225290825474075973033905029296875;0.32557089580899367664557075841003097593784332275390625]
      mask Display: e = 0.06;c1 = [120 150 230]/255;c2 = ([120 150 230]+0)/383;c3 = ([120 150 230]+128)/383;patch([0 1 1 0],[0 0 1 1],c1);patch([0 1 1 1-e 1-e 0+e],[0 0 1 1-e 0+e 0+e],c2);patch([0 0 1 1-e 0+e 0+e],[0 1 1 1-e 1-e 0+e],c3);plot([0 1 1 0 0],[0 0 1 1 0]);disp('Weights');
  "IW{1,1}(9,:)'" : Constant  Value=[-0.220653591087006162307915246856282465159893035888671875;1.2430267736595876915117742100846953690052032470703125;-0.6481087415921036321009296443662606179714202880859375;1.3983883992961183562186988638131879270076751708984375;-1.072074538433060109099415058153681457042694091796875;-0.267444379464151504866009645411395467817783355712890625;-0.6571027188807623264921176087227649986743927001953125]
      mask Display: e = 0.06;c1 = [120 150 230]/255;c2 = ([120 150 230]+0)/383;c3 = ([120 150 230]+128)/383;patch([0 1 1 0],[0 0 1 1],c1);patch([0 1 1 1-e 1-e 0+e],[0 0 1 1-e 0+e 0+e],c2);patch([0 0 1 1-e 0+e 0+e],[0 1 1 1-e 1-e 0+e],c3);plot([0 1 1 0 0],[0 0 1 1 0]);disp('Weights');
  Mux : Mux  Inputs=57
      mask Display: e = 0.06;c1 = [120 150 230]/255;c2 = ([120 150 230]+0)/383;c3 = ([120 150 230]+128)/383;patch([0 1 1 0],[0 0 1 1],c1);patch([0 1 1 1-e 1-e 0+e],[0 0 1 1-e 0+e 0+e],c2);patch([0 0 1 1-e 0+e 0+e],[0 1 1 1-e 1-e 0+e],c3);plot([0 1 1 0 0],[0 0 1 1 0]);disp('Mux');
  dotprod{1..57} (57 alike) : neural/Weight Functions/dotprod
  "iz{1,1}" : Outport
      mask Display: e = 0.06;c1 = [120 230 180]/255;c2 = ([120 230 180]+0)/(256+128);c3 = ([120 230 180]+128)/(256+128);patch([0 1 1 0],[0 0 1 1],c1);patch([0 1 1 1-e 1-e 0+e],[0 0 1 1-e 0+e 0+e],c2);patch([0 0 1 1-e 0+e 0+e],[0 1 1 1-e 1-e 0+e],c3);plot([0 1 1 0 0],[0 0 1 1 0]);
  wires:
  "IW{1,1}(1,:)'"/1 -> dotprod1/1
  "pd{1,1}"/1 -> dotprod1/2, dotprod2/2, dotprod3/2, dotprod4/2, dotprod5/2, dotprod6/2, dotprod7/2, dotprod8/2, dotprod9/2, dotprod10/2, dotprod11/2, dotprod12/2, dotprod13/2, dotprod14/2, dotprod15/2, dotprod16/2, dotprod17/2, dotprod18/2, dotprod19/2, dotprod20/2, dotprod21/2, dotprod22/2, dotprod23/2, dotprod24/2, dotprod25/2, dotprod26/2, dotprod27/2, dotprod28/2, dotprod29/2, dotprod30/2, dotprod31/2, dotprod32/2, dotprod33/2, dotprod34/2, dotprod35/2, dotprod36/2, dotprod37/2, dotprod38/2, dotprod39/2, dotprod40/2, dotprod41/2, dotprod42/2, dotprod43/2, dotprod44/2, dotprod45/2, dotprod46/2, dotprod47/2, dotprod48/2, dotprod49/2, dotprod50/2, dotprod51/2, dotprod52/2, dotprod53/2, dotprod54/2, dotprod55/2, dotprod56/2, dotprod57/2
  dotprod1/1 -> Mux/1
  "IW{1,1}(2,:)'"/1 -> dotprod2/1
  dotprod2/1 -> Mux/2
  "IW{1,1}(3,:)'"/1 -> dotprod3/1
  dotprod3/1 -> Mux/3
  "IW{1,1}(4,:)'"/1 -> dotprod4/1
  dotprod4/1 -> Mux/4
  "IW{1,1}(5,:)'"/1 -> dotprod5/1
  dotprod5/1 -> Mux/5
  "IW{1,1}(6,:)'"/1 -> dotprod6/1
  dotprod6/1 -> Mux/6
  "IW{1,1}(7,:)'"/1 -> dotprod7/1
  dotprod7/1 -> Mux/7
  "IW{1,1}(8,:)'"/1 -> dotprod8/1
  dotprod8/1 -> Mux/8
  "IW{1,1}(9,:)'"/1 -> dotprod9/1
  dotprod9/1 -> Mux/9
  "IW{1,1}(10,:)'"/1 -> dotprod10/1
  dotprod10/1 -> Mux/10
  "IW{1,1}(11,:)'"/1 -> dotprod11/1
  dotprod11/1 -> Mux/11
  "IW{1,1}(12,:)'"/1 -> dotprod12/1
  dotprod12/1 -> Mux/12
  "IW{1,1}(13,:)'"/1 -> dotprod13/1
  dotprod13/1 -> Mux/13
  "IW{1,1}(14,:)'"/1 -> dotprod14/1
  dotprod14/1 -> Mux/14
  "IW{1,1}(15,:)'"/1 -> dotprod15/1
  dotprod15/1 -> Mux/15
  "IW{1,1}(16,:)'"/1 -> dotprod16/1
  dotprod16/1 -> Mux/16
  "IW{1,1}(17,:)'"/1 -> dotprod17/1
  dotprod17/1 -> Mux/17
  "IW{1,1}(18,:)'"/1 -> dotprod18/1
  dotprod18/1 -> Mux/18
  "IW{1,1}(19,:)'"/1 -> dotprod19/1
  dotprod19/1 -> Mux/19
  "IW{1,1}(20,:)'"/1 -> dotprod20/1
  dotprod20/1 -> Mux/20
  "IW{1,1}(21,:)'"/1 -> dotprod21/1
  dotprod21/1 -> Mux/21
  "IW{1,1}(22,:)'"/1 -> dotprod22/1
  dotprod22/1 -> Mux/22
  "IW{1,1}(23,:)'"/1 -> dotprod23/1
  dotprod23/1 -> Mux/23
  "IW{1,1}(24,:)'"/1 -> dotprod24/1
  dotprod24/1 -> Mux/24
  "IW{1,1}(25,:)'"/1 -> dotprod25/1
  dotprod25/1 -> Mux/25
  "IW{1,1}(26,:)'"/1 -> dotprod26/1
  dotprod26/1 -> Mux/26
  "IW{1,1}(27,:)'"/1 -> dotprod27/1
  dotprod27/1 -> Mux/27
  "IW{1,1}(28,:)'"/1 -> dotprod28/1
  dotprod28/1 -> Mux/28
  "IW{1,1}(29,:)'"/1 -> dotprod29/1
  dotprod29/1 -> Mux/29
  "IW{1,1}(30,:)'"/1 -> dotprod30/1
  dotprod30/1 -> Mux/30
  "IW{1,1}(31,:)'"/1 -> dotprod31/1
  dotprod31/1 -> Mux/31
  "IW{1,1}(32,:)'"/1 -> dotprod32/1
  dotprod32/1 -> Mux/32
  "IW{1,1}(33,:)'"/1 -> dotprod33/1
  dotprod33/1 -> Mux/33
  "IW{1,1}(34,:)'"/1 -> dotprod34/1
  dotprod34/1 -> Mux/34
  "IW{1,1}(35,:)'"/1 -> dotprod35/1
  dotprod35/1 -> Mux/35
  "IW{1,1}(36,:)'"/1 -> dotprod36/1
  dotprod36/1 -> Mux/36
  "IW{1,1}(37,:)'"/1 -> dotprod37/1
  dotprod37/1 -> Mux/37
  "IW{1,1}(38,:)'"/1 -> dotprod38/1
  dotprod38/1 -> Mux/38
  "IW{1,1}(39,:)'"/1 -> dotprod39/1
  dotprod39/1 -> Mux/39
  "IW{1,1}(40,:)'"/1 -> dotprod40/1
  dotprod40/1 -> Mux/40
  "IW{1,1}(41,:)'"/1 -> dotprod41/1
  dotprod41/1 -> Mux/41
  "IW{1,1}(42,:)'"/1 -> dotprod42/1
  dotprod42/1 -> Mux/42
  "IW{1,1}(43,:)'"/1 -> dotprod43/1
  dotprod43/1 -> Mux/43
  "IW{1,1}(44,:)'"/1 -> dotprod44/1
  dotprod44/1 -> Mux/44
  "IW{1,1}(45,:)'"/1 -> dotprod45/1
  dotprod45/1 -> Mux/45
  "IW{1,1}(46,:)'"/1 -> dotprod46/1
  dotprod46/1 -> Mux/46
  "IW{1,1}(47,:)'"/1 -> dotprod47/1
  dotprod47/1 -> Mux/47
  "IW{1,1}(48,:)'"/1 -> dotprod48/1
  dotprod48/1 -> Mux/48
  "IW{1,1}(49,:)'"/1 -> dotprod49/1
  dotprod49/1 -> Mux/49
  "IW{1,1}(50,:)'"/1 -> dotprod50/1
  dotprod50/1 -> Mux/50
  "IW{1,1}(51,:)'"/1 -> dotprod51/1
  dotprod51/1 -> Mux/51
  "IW{1,1}(52,:)'"/1 -> dotprod52/1
  dotprod52/1 -> Mux/52
  "IW{1,1}(53,:)'"/1 -> dotprod53/1
  dotprod53/1 -> Mux/53
  "IW{1,1}(54,:)'"/1 -> dotprod54/1
  dotprod54/1 -> Mux/54
  "IW{1,1}(55,:)'"/1 -> dotprod55/1
  dotprod55/1 -> Mux/55
  "IW{1,1}(56,:)'"/1 -> dotprod56/1
  dotprod56/1 -> Mux/56
  "IW{1,1}(57,:)'"/1 -> dotprod57/1
  dotprod57/1 -> Mux/57
  Mux/1 -> "iz{1,1}"/1

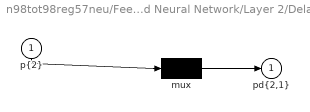
== system n98tot98reg57neu/Feed-Forward Neural Network/Layer 2/Delays 1 ==
  "p{2}" : Inport  PortDimensions=57
      mask Display: e = 0.06;c1 = [120 230 180]/255;c2 = ([120 230 180]+0)/(256+128);c3 = ([120 230 180]+128)/(256+128);patch([0 1 1 0],[0 0 1 1],c1);patch([0 1 1 1-e 1-e 0+e],[0 0 1 1-e 0+e 0+e],c2);patch([0 0 1 1-e 0+e 0+e],[0 1 1 1-e 1-e 0+e],c3);plot([0 1 1 0 0],[0 0 1 1 0]);
  mux : Mux  Inputs=1
      mask Display: e = 0.06;c1 = [120 150 230]/255;c2 = ([120 150 230]+0)/383;c3 = ([120 150 230]+128)/383;patch([0 1 1 0],[0 0 1 1],c1);patch([0 1 1 1-e 1-e 0+e],[0 0 1 1-e 0+e 0+e],c2);patch([0 0 1 1-e 0+e 0+e],[0 1 1 1-e 1-e 0+e],c3);plot([0 1 1 0 0],[0 0 1 1 0]);disp('Mux')
  "pd{2,1}" : Outport
      mask Display: e = 0.06;c1 = [120 230 180]/255;c2 = ([120 230 180]+0)/(256+128);c3 = ([120 230 180]+128)/(256+128);patch([0 1 1 0],[0 0 1 1],c1);patch([0 1 1 1-e 1-e 0+e],[0 0 1 1-e 0+e 0+e],c2);patch([0 0 1 1-e 0+e 0+e],[0 1 1 1-e 1-e 0+e],c3);plot([0 1 1 0 0],[0 0 1 1 0]);
  wires:
  "p{2}"/1 -> mux/1
  mux/1 -> "pd{2,1}"/1
